simulink model "uas_sim"  (R2020b)
settings: Solver=VariableStepAuto  StartTime=0.0  StopTime=10.0  RelTol=1e-3  SampleTimeConstraint=STIndependent
undefined symbols (not defined in the file): Aircraft, datetime, datevec, Earth, Env, InitCond, WGS84
libraries: aerolibconvert2 x8, simulink x8, aerolibadyn x3, aerolibasang x3, aerolibtransform2 x2, aerolibatmos2 x1, sharedutil x1, aerolibbdyn x1, shared6dof x1, aerolibgravity2 x1
(part 2 of 2)

== system uas_sim/Flight Management Unit/Sensor Models/IMU/Accelerometer ==
  Body Accel [m/s/s] : Inport  PortDimensions=3
  Gravitational Accel in Body Frame [m/s/s] : Inport  Port=2  PortDimensions=3
  Add : Sum  Inputs=+++
  Band-Limited White Noise : simulink/Sources/Band-Limited White Noise  Cov=Aircraft.Sensors.Imu.Accel.noise_mps2  Ts=0.1  seed=[23341]
  Constant : Constant  Value=Aircraft.Sensors.Imu.Accel.bias_mps2  VectorParams1D=off
  Constant1 : Constant  Value=Aircraft.Sensors.Imu.Accel.scale_factor
  Product : Product  Multiplication=Matrix(*)
  Reshape : Reshape  OutputDimensionality=Column vector (2-D)
  Reshape1 : Reshape  OutputDimensionality=Column vector (2-D)
  Reshape2 : Reshape
  Saturation : Saturate  UpperLimit=Aircraft.Sensors.Imu.Accel.upper_limit_mps2  LowerLimit=Aircraft.Sensors.Imu.Accel.lower_limit_mps2
  Subtract : Sum  Inputs=+-
  Accelerometer [m/s/s] : Outport  PortDimensions=3
  wires:
  Add/1 -> Saturation/1
  Band-Limited White Noise/1 -> Add/1
  Product/1 -> Add/3
  Constant/1 -> Add/2
  Constant1/1 -> Product/1
  Subtract/1 -> Product/2
  Reshape/1 -> Subtract/2
  Gravitational Accel in Body Frame [m/s/s]/1 -> Reshape/1
  Reshape1/1 -> Subtract/1
  Body Accel [m/s/s]/1 -> Reshape1/1
  Saturation/1 -> Reshape2/1
  Reshape2/1 -> Accelerometer [m/s/s]/1

== system uas_sim/Flight Management Unit/Sensor Models/IMU/Gyro ==
  Body Rotational Rate [rad/s] : Inport  PortDimensions=3
  Body Accel [m/s/s] : Inport  Port=2  PortDimensions=3
  Add1 : Sum  Inputs=++++
  Band-Limited White Noise : simulink/Sources/Band-Limited White Noise  Cov=Aircraft.Sensors.Imu.Gyro.noise_radps  Ts=0.1  seed=[23341]  VectorParams1D=off
  Constant1 : Constant  Value=Aircraft.Sensors.Imu.Gyro.bias_radps  VectorParams1D=off
  Constant2 : Constant  Value=Aircraft.Sensors.Imu.Gyro.accel_sens_radps
  Constant3 : Constant  Value=Aircraft.Sensors.Imu.Gyro.scale_factor  VectorParams1D=off
  Product : Product
  Product1 : Product  Multiplication=Matrix(*)
  Reshape : Reshape  OutputDimensionality=Column vector (2-D)
  Reshape1 : Reshape  OutputDimensionality=Column vector (2-D)
  Reshape2 : Reshape
  Saturation : Saturate  UpperLimit=Aircraft.Sensors.Imu.Gyro.upper_limit_radps  LowerLimit=Aircraft.Sensors.Imu.Gyro.lower_limit_radps
  Gyro [rad/s] : Outport  PortDimensions=3
  wires:
  Constant3/1 -> Product1/1
  Constant2/1 -> Product/1
  Add1/1 -> Saturation/1
  Constant1/1 -> Add1/3
  Product1/1 -> Add1/4
  Band-Limited White Noise/1 -> Add1/2
  Body Rotational Rate [rad/s]/1 -> Reshape/1
  Reshape/1 -> Product1/2
  Body Accel [m/s/s]/1 -> Product/2
  Product/1 -> Reshape1/1
  Reshape1/1 -> Add1/1
  Reshape2/1 -> Gyro [rad/s]/1
  Saturation/1 -> Reshape2/1

== system uas_sim/Flight Management Unit/Sensor Models/IMU/Magnetometer ==
  Body Magnetic Field [uT] : Inport  PortDimensions=3
  Add2 : Sum  Inputs=+++
  Band-Limited White Noise : simulink/Sources/Band-Limited White Noise  Cov=Aircraft.Sensors.Imu.Mag.noise_ut  Ts=0.1  seed=[23341]
  Constant1 : Constant  Value=Aircraft.Sensors.Imu.Mag.scale_factor  VectorParams1D=off
  Constant2 : Constant  Value=Aircraft.Sensors.Imu.Mag.bias_ut
  Product : Product  Multiplication=Matrix(*)
  Reshape : Reshape  OutputDimensionality=Column vector (2-D)
  Reshape1 : Reshape
  Saturation : Saturate  UpperLimit=Aircraft.Sensors.Imu.Mag.upper_limit_ut  LowerLimit=Aircraft.Sensors.Imu.Mag.lower_limit_ut
  Magnetometer [uT] : Outport  PortDimensions=3
  wires:
  Body Magnetic Field [uT]/1 -> Reshape/1
  Band-Limited White Noise/1 -> Add2/1
  Add2/1 -> Saturation/1
  Constant2/1 -> Add2/2
  Constant1/1 -> Product/1
  Reshape/1 -> Product/2
  Saturation/1 -> Reshape1/1
  Reshape1/1 -> Magnetometer [uT]/1
  Product/1 -> Add2/3

== system uas_sim/Flight Management Unit/Vehicle Management System/Sensor Data Mapping/Air Data Mapping ==
  Virtual : Inport
  Bus Creator : BusCreator  Inputs=2  OutDataTypeStr=Bus: AirData
      settings: InheritFromInputs=off
  Bus Selector : BusSelector  OutputSignals=Static Pressure [Pa],Differential Pressure [Pa]
  Data Type Conversion1 : DataTypeConversion  OutDataTypeStr=single
  Data Type Conversion6 : DataTypeConversion  OutDataTypeStr=single
  Non-virtual : Outport  OutDataTypeStr=Bus: AirData
  wires:
  Virtual/1 -> Bus Selector/1
  Bus Creator/1 -> Non-virtual/1
  Bus Selector/2 -> Data Type Conversion1/1  "<Differential Pressure [Pa]>"
  Bus Selector/1 -> Data Type Conversion6/1  "<Static Pressure [Pa]>"
  Data Type Conversion6/1 -> Bus Creator/1  "static_pres_pa"
  Data Type Conversion1/1 -> Bus Creator/2  "diff_pres_pa"

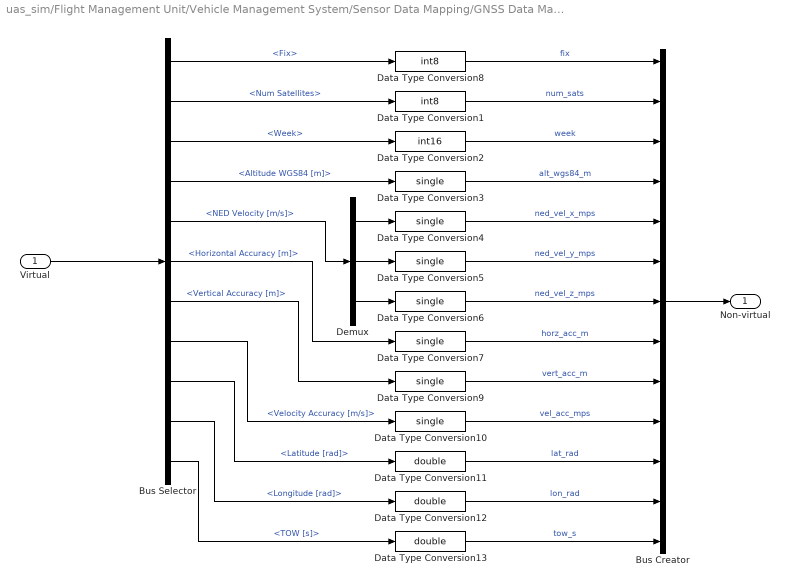
== system uas_sim/Flight Management Unit/Vehicle Management System/Sensor Data Mapping/GNSS Data Mapping ==
  Virtual : Inport
  Bus Creator : BusCreator  Inputs=13  OutDataTypeStr=Bus: GnssData
      settings: InheritFromInputs=off
  Bus Selector : BusSelector  OutputSignals=Fix,Num Satellites,Week,Altitude WGS84 [m],NED Velocity [m/s],Horizontal Accuracy [m],Vertical Accuracy [m],Velocity Accuracy [m/s],Latitude [rad],Longitude [rad],TOW [s]
  Data Type Conversion1 : DataTypeConversion  OutDataTypeStr=int8
  Data Type Conversion{3..7,9..10} (7 alike) : DataTypeConversion  OutDataTypeStr=single
  Data Type Conversion11 : DataTypeConversion  OutDataTypeStr=double
  Data Type Conversion12 : DataTypeConversion  OutDataTypeStr=double
  Data Type Conversion13 : DataTypeConversion  OutDataTypeStr=double
  Data Type Conversion2 : DataTypeConversion  OutDataTypeStr=int16
  Data Type Conversion8 : DataTypeConversion  OutDataTypeStr=int8
  Demux : Demux  Outputs=3
  Non-virtual : Outport  OutDataTypeStr=Bus: GnssData
  wires:
  Bus Creator/1 -> Non-virtual/1
  Virtual/1 -> Bus Selector/1
  Bus Selector/1 -> Data Type Conversion8/1  "<Fix>"
  Data Type Conversion8/1 -> Bus Creator/1  "fix"
  Bus Selector/2 -> Data Type Conversion1/1  "<Num Satellites>"
  Data Type Conversion1/1 -> Bus Creator/2  "num_sats"
  Data Type Conversion2/1 -> Bus Creator/3  "week"
  Bus Selector/3 -> Data Type Conversion2/1  "<Week>"
  Bus Selector/4 -> Data Type Conversion3/1  "<Altitude WGS84 [m]>"
  Data Type Conversion3/1 -> Bus Creator/4  "alt_wgs84_m"
  Demux/2 -> Data Type Conversion5/1
  Demux/1 -> Data Type Conversion4/1
  Demux/3 -> Data Type Conversion6/1
  Bus Selector/5 -> Demux/1  "<NED Velocity [m/s]>"
  Data Type Conversion4/1 -> Bus Creator/5  "ned_vel_x_mps"
  Data Type Conversion5/1 -> Bus Creator/6  "ned_vel_y_mps"
  Data Type Conversion6/1 -> Bus Creator/7  "ned_vel_z_mps"
  Data Type Conversion7/1 -> Bus Creator/8  "horz_acc_m"
  Bus Selector/6 -> Data Type Conversion7/1  "<Horizontal Accuracy [m]>"
  Data Type Conversion9/1 -> Bus Creator/9  "vert_acc_m"
  Data Type Conversion10/1 -> Bus Creator/10  "vel_acc_mps"
  Data Type Conversion11/1 -> Bus Creator/11  "lat_rad"
  Data Type Conversion12/1 -> Bus Creator/12  "lon_rad"
  Data Type Conversion13/1 -> Bus Creator/13  "tow_s"
  Bus Selector/11 -> Data Type Conversion13/1  "<TOW [s]>"
  Bus Selector/10 -> Data Type Conversion12/1  "<Longitude [rad]>"
  Bus Selector/9 -> Data Type Conversion11/1  "<Latitude [rad]>"
  Bus Selector/8 -> Data Type Conversion10/1  "<Velocity Accuracy [m/s]>"
  Bus Selector/7 -> Data Type Conversion9/1  "<Vertical Accuracy [m]>"

== system uas_sim/Flight Management Unit/Vehicle Management System/Sensor Data Mapping/IMU Data Mapping ==
  Virtual : Inport
  Bus Creator : BusCreator  Inputs=9  OutDataTypeStr=Bus: ImuData
      settings: InheritFromInputs=off
  Bus Selector : BusSelector  OutputSignals=Accelerometer [m/s/s],Gyro [rad/s],Magnetometer [uT]
  Data Type Conversion{1..9} (9 alike) : DataTypeConversion  OutDataTypeStr=single
  Demux : Demux  Outputs=3
  Demux1 : Demux  Outputs=3
  Demux2 : Demux  Outputs=3
  Non-virtual : Outport  OutDataTypeStr=Bus: ImuData
  wires:
  Virtual/1 -> Bus Selector/1
  Bus Creator/1 -> Non-virtual/1
  Demux/1 -> Data Type Conversion8/1
  Data Type Conversion8/1 -> Bus Creator/1  "accel_x_mps2"
  Demux/2 -> Data Type Conversion1/1
  Data Type Conversion1/1 -> Bus Creator/2  "accel_y_mps2"
  Demux/3 -> Data Type Conversion2/1
  Data Type Conversion2/1 -> Bus Creator/3  "accel_z_mps2"
  Data Type Conversion4/1 -> Bus Creator/6  "gyro_z_radps"
  Demux1/3 -> Data Type Conversion4/1
  Data Type Conversion3/1 -> Bus Creator/5  "gyro_y_radps"
  Demux1/2 -> Data Type Conversion3/1
  Data Type Conversion5/1 -> Bus Creator/4  "gyro_x_radps"
  Demux1/1 -> Data Type Conversion5/1
  Demux2/1 -> Data Type Conversion9/1
  Data Type Conversion9/1 -> Bus Creator/7  "mag_x_ut"
  Demux2/2 -> Data Type Conversion6/1
  Data Type Conversion6/1 -> Bus Creator/8  "mag_y_ut"
  Demux2/3 -> Data Type Conversion7/1
  Data Type Conversion7/1 -> Bus Creator/9  "mag_z-ut"
  Bus Selector/1 -> Demux/1  "<Accelerometer [m/s/s]>"
  Bus Selector/2 -> Demux1/1  "<Gyro [rad/s]>"
  Bus Selector/3 -> Demux2/1  "<Magnetometer [uT]>"

== system uas_sim/Vehicle/Forces and Moments/Aerodynamic/Aerodynamic Forces and Moments Coef Axis Variant ==
  Coef : Inport
  Dynamic Pressure [Pa] : Inport  Port=2
  Body Velocity [m/s] : Inport  Port=3
  Body Axis Coef : Subsystem  VariantControl=Aircraft.Aero.axis == 3
  Stability Axis Coef : Subsystem  VariantControl=Aircraft.Aero.axis == 2
  Wind Axis Coef : Subsystem  VariantControl=Aircraft.Aero.axis == 1
  Fxyz Mxyz : Outport

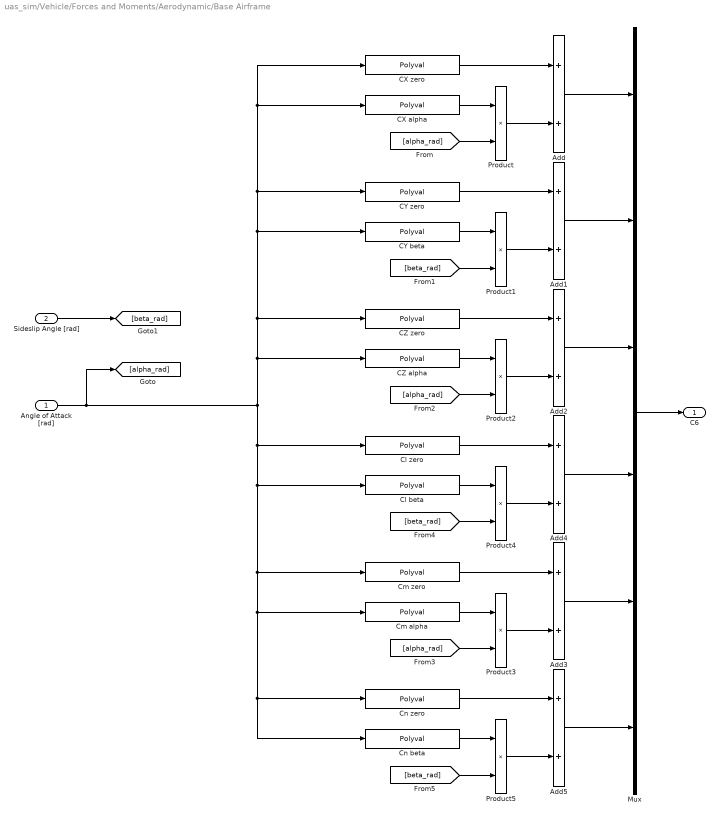
== system uas_sim/Vehicle/Forces and Moments/Aerodynamic/Base Airframe ==
  Angle of Attack [rad] : Inport
  Sideslip Angle [rad] : Inport  Port=2
  Add{,1..5} (6 alike) : Sum
  CX alpha : Polyval  Coefs=Aircraft.Aero.CX.alpha
  CX zero : Polyval  Coefs=Aircraft.Aero.CX.zero
  CY beta : Polyval  Coefs=Aircraft.Aero.CY.beta
  CY zero : Polyval  Coefs=Aircraft.Aero.CY.zero
  CZ alpha : Polyval  Coefs=Aircraft.Aero.CZ.alpha
  CZ zero : Polyval  Coefs=Aircraft.Aero.CZ.zero
  Cl beta : Polyval  Coefs=Aircraft.Aero.Cl.beta
  Cl zero : Polyval  Coefs=Aircraft.Aero.Cl.zero
  Cm alpha : Polyval  Coefs=Aircraft.Aero.Cm.alpha
  Cm zero : Polyval  Coefs=Aircraft.Aero.Cm.zero
  Cn beta : Polyval  Coefs=Aircraft.Aero.Cn.beta
  Cn zero : Polyval  Coefs=Aircraft.Aero.Cn.zero
  Mux : Mux  Inputs=6
  Product{,1..5} (6 alike) : Product
  C6 : Outport
  wires:
  Product/1 -> Add/2
  Add/1 -> Mux/1
  CX alpha/1 -> Product/1
  CX zero/1 -> Add/1
  Sideslip Angle [rad]/1 -> [beta_rad]
  [alpha_rad] -> Product/2
  Mux/1 -> C6/1
  [beta_rad] -> Product1/2
  CY zero/1 -> Add1/1
  CY beta/1 -> Product1/1
  Product1/1 -> Add1/2
  Add1/1 -> Mux/2
  CZ zero/1 -> Add2/1
  CZ alpha/1 -> Product2/1
  Add2/1 -> Mux/3
  Product2/1 -> Add2/2
  Product3/1 -> Add3/2
  Add3/1 -> Mux/5
  Cm alpha/1 -> Product3/1
  Cm zero/1 -> Add3/1
  [alpha_rad] -> Product2/2
  [alpha_rad] -> Product3/2
  Add4/1 -> Mux/4
  Product4/1 -> Add4/2
  Cl beta/1 -> Product4/1
  Cl zero/1 -> Add4/1
  [beta_rad] -> Product4/2
  [beta_rad] -> Product5/2
  Cn zero/1 -> Add5/1
  Cn beta/1 -> Product5/1
  Product5/1 -> Add5/2
  Add5/1 -> Mux/6
  Angle of Attack [rad]/1 -> [alpha_rad], Cl zero/1, Cl beta/1, Cm zero/1, Cm alpha/1, Cn zero/1, Cn beta/1, CZ alpha/1, CZ zero/1, CY beta/1, CY zero/1, CX alpha/1, CX zero/1

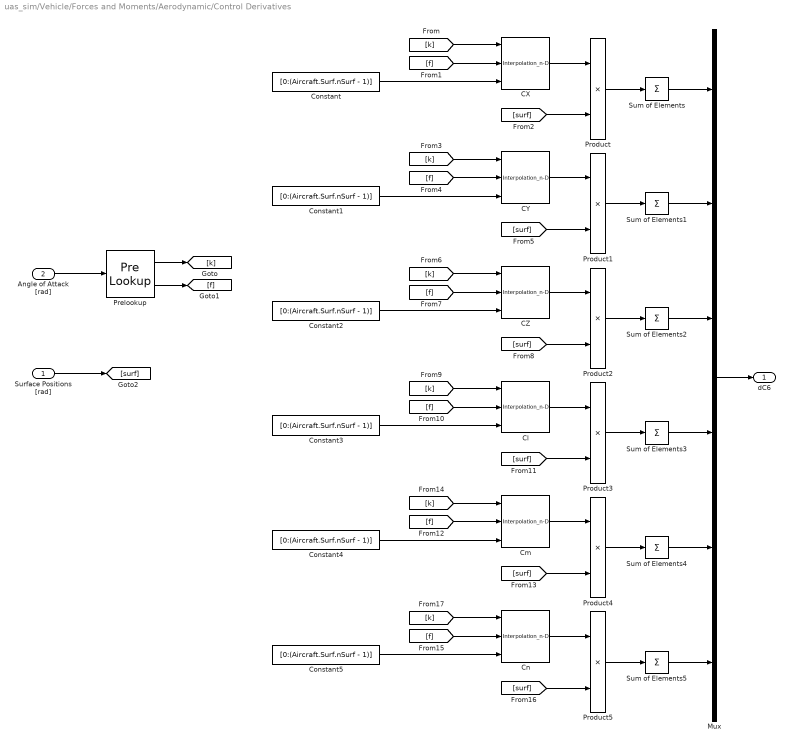
== system uas_sim/Vehicle/Forces and Moments/Aerodynamic/Control Derivatives ==
  Surface Positions [rad] : Inport
  Angle of Attack [rad] : Inport  Port=2
  CX : Interpolation_n-D  Table=Aircraft.Aero.CX.surf  DiagnosticForOutOfRangeInput=Warning  NumSelectionDims=1  InternalRulePriority=Speed
      settings: InputPortMap=u0,u1,u2
  CY : Interpolation_n-D  Table=Aircraft.Aero.CY.surf  DiagnosticForOutOfRangeInput=Warning  NumSelectionDims=1  InternalRulePriority=Speed
      settings: InputPortMap=u0,u1,u2
  CZ : Interpolation_n-D  Table=Aircraft.Aero.CZ.surf  DiagnosticForOutOfRangeInput=Warning  NumSelectionDims=1  InternalRulePriority=Speed
      settings: InputPortMap=u0,u1,u2
  Cl : Interpolation_n-D  Table=Aircraft.Aero.Cl.surf  DiagnosticForOutOfRangeInput=Warning  NumSelectionDims=1  InternalRulePriority=Speed
      settings: InputPortMap=u0,u1,u2
  Cm : Interpolation_n-D  Table=Aircraft.Aero.Cm.surf  DiagnosticForOutOfRangeInput=Warning  NumSelectionDims=1  InternalRulePriority=Speed
      settings: InputPortMap=u0,u1,u2
  Cn : Interpolation_n-D  Table=Aircraft.Aero.Cn.surf  DiagnosticForOutOfRangeInput=Warning  NumSelectionDims=1  InternalRulePriority=Speed
      settings: InputPortMap=u0,u1,u2
  Constant{,1..5} (6 alike) : Constant  Value=[0:(Aircraft.Surf.nSurf - 1)]
  Mux : Mux  Inputs=6
  Prelookup : PreLookup  BreakpointsData=Aircraft.Aero.CntrlEff.alpha  ExtrapMethod=Linear
  Product{,1..5} (6 alike) : Product
  Sum of Elements{,1..5} (6 alike) : Sum  Inputs=+
  dC6 : Outport
  wires:
  [k] -> Cm/1
  CY/1 -> Product1/1
  [f] -> Cn/2
  Product5/1 -> Sum of Elements5/1
  [surf] -> Product5/2
  Constant4/1 -> Cm/3
  Sum of Elements1/1 -> Mux/2
  [k] -> Cn/1
  Sum of Elements5/1 -> Mux/6
  Constant3/1 -> Cl/3
  [surf] -> Product3/2
  [k] -> Cl/1
  [f] -> Cl/2
  Constant2/1 -> CZ/3
  [k] -> CZ/1
  [surf] -> Product2/2
  Cl/1 -> Product3/1
  CZ/1 -> Product2/1
  Product2/1 -> Sum of Elements2/1
  Product3/1 -> Sum of Elements3/1
  Product1/1 -> Sum of Elements1/1
  Product/1 -> Sum of Elements/1
  [k] -> CY/1
  [f] -> CY/2
  Constant1/1 -> CY/3
  Constant/1 -> CX/3
  Cm/1 -> Product4/1
  [k] -> CX/1
  [surf] -> Product/2
  Prelookup/2 -> [f]
  Mux/1 -> dC6/1
  Prelookup/1 -> [k]
  Product4/1 -> Sum of Elements4/1
  Cn/1 -> Product5/1
  Angle of Attack [rad]/1 -> Prelookup/1
  Surface Positions [rad]/1 -> [surf]
  [f] -> CZ/2
  [f] -> Cm/2
  Sum of Elements2/1 -> Mux/3
  CX/1 -> Product/1
  [f] -> CX/2
  Constant5/1 -> Cn/3
  [surf] -> Product4/2
  Sum of Elements/1 -> Mux/1
  Sum of Elements4/1 -> Mux/5
  [surf] -> Product1/2
  Sum of Elements3/1 -> Mux/4

== system uas_sim/Vehicle/Forces and Moments/Aerodynamic/Dynamic Derivatives ==
  note: Divide by zero protection
  Airspeed [m/s] : Inport
  Body Rotational Rate [rad/s] : Inport  Port=2
  Angle of Attack [rad] : Inport  Port=3
  Add : Sum  Inputs=+++
  Constant : Constant  Value=Aircraft.Geom.b_m
  Constant1 : Constant  Value=Aircraft.Geom.c_m
  Constant2 : Constant  Value=Aircraft.Geom.b_m
  Demux : Demux  Outputs=3
  Divide : Product  Inputs=*/
  Gain : Gain  Gain=2
  Mux : Mux  Inputs=3
  Pitch Rate : Subsystem
  Product : Product
  Roll Rate : Subsystem
  Saturation : Saturate  UpperLimit=inf  LowerLimit=1e-3
  Yaw Rate : Subsystem
  dC6 : Outport
  wires:
  Constant/1 -> Mux/1
  Body Rotational Rate [rad/s]/1 -> Product/1
  Mux/1 -> Product/2
  Airspeed [m/s]/1 -> Gain/1
  Gain/1 -> Saturation/1
  Product/1 -> Divide/1
  Saturation/1 -> Divide/2
  Divide/1 -> Demux/1
  Demux/1 -> Roll Rate/2(p_hat)
  Demux/2 -> Pitch Rate/2(q_hat)
  Demux/3 -> Yaw Rate/2(r_hat)
  Angle of Attack [rad]/1 -> Yaw Rate/1(Angle of Attack [rad]), Pitch Rate/1(Angle of Attack [rad]), Roll Rate/1(Angle of Attack [rad])
  Roll Rate/1(dC6) -> Add/1
  Pitch Rate/1(dC6) -> Add/2
  Yaw Rate/1(dC6) -> Add/3
  Constant2/1 -> Mux/3
  Constant1/1 -> Mux/2
  Add/1 -> dC6/1

== system uas_sim/Vehicle/Forces and Moments/Propulsive/Motor ==
  note: RPM to rad/s
  Voltage [V] : Inport
  Motor Rotation Rate [rad/s] : Inport  Port=2
  Constant : Constant  Value=Aircraft.Motor.kv
  Constant1 : Constant  Value=Aircraft.Motor.io
  Divide : Product  Inputs=*/
  Divide2 : Product  Inputs=*/
  Gain : Gain  Gain=1/Aircraft.Motor.r
  Gain2 : Gain  Gain=2 * pi / 60
  Subtract : Sum  Inputs=+-
  Subtract1 : Sum  Inputs=+-
  Torque [N-m] : Outport
  wires:
  Gain2/1 -> [KvSI], Divide/2
  [KvSI] -> Divide2/2
  Constant1/1 -> Subtract1/2
  Motor Rotation Rate [rad/s]/1 -> Divide/1
  Divide/1 -> Subtract/2
  Constant/1 -> Gain2/1
  Gain/1 -> Subtract1/1
  Subtract1/1 -> Divide2/1
  Voltage [V]/1 -> Subtract/1
  Divide2/1 -> Torque [N-m]/1
  Subtract/1 -> Gain/1

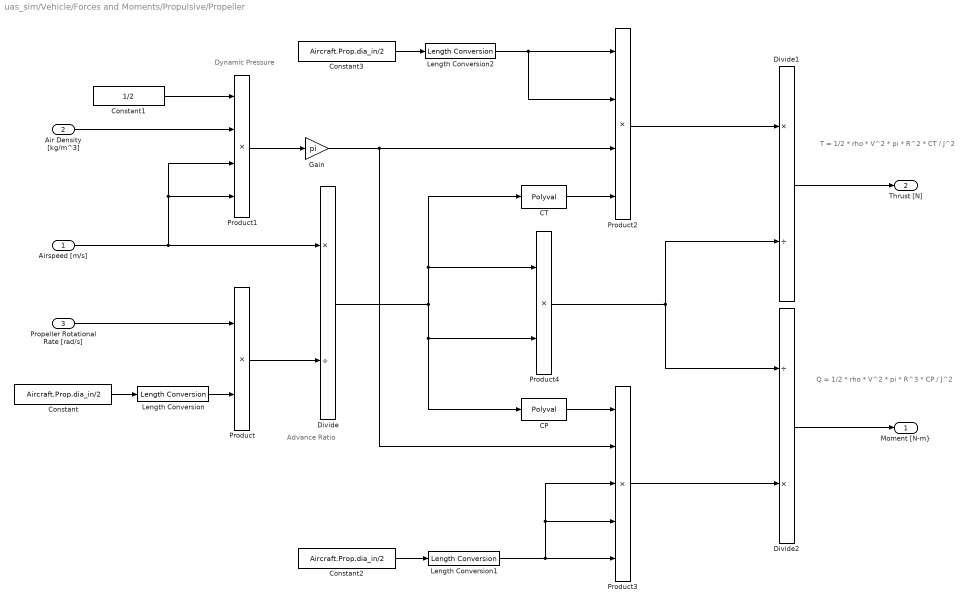
== system uas_sim/Vehicle/Forces and Moments/Propulsive/Propeller ==
  note: Dynamic Pressure
  note: Q = 1/2 * rho * V^2 * pi * R^3 * CP / J^2
  note: T = 1/2 * rho * V^2 * pi * R^2 * CT / J^2
  note: Advance Ratio
  Airspeed [m/s] : Inport
  Air Density [kg/m^3] : Inport  Port=2
  Propeller Rotational Rate [rad/s] : Inport  Port=3
  CP : Polyval  Coefs=Aircraft.prop.cp
  CT : Polyval  Coefs=Aircraft.prop.ct
  Constant : Constant  Value=Aircraft.Prop.dia_in/2
  Constant1 : Constant  Value=1/2
  Constant2 : Constant  Value=Aircraft.Prop.dia_in/2
  Constant3 : Constant  Value=Aircraft.Prop.dia_in/2
  Divide : Product  Inputs=*/
  Divide1 : Product  Inputs=*/
  Divide2 : Product  Inputs=/*
  Gain : Gain  Gain=pi
  Length Conversion : aerolibconvert2/Length Conversion  IU=in  OU=m
  Length Conversion1 : aerolibconvert2/Length Conversion  IU=in  OU=m
  Length Conversion2 : aerolibconvert2/Length Conversion  IU=in  OU=m
  Product : Product
  Product1 : Product  Inputs=4
  Product2 : Product  Inputs=4
  Product3 : Product  Inputs=5
  Product4 : Product
  "Moment [N-m}" : Outport
  Thrust [N] : Outport  Port=2
  wires:
  Divide2/1 -> "Moment [N-m}"/1
  Length Conversion/1 -> Product/2
  Product4/1 -> Divide2/1, Divide1/2
  Constant2/1 -> Length Conversion1/1
  Airspeed [m/s]/1 -> Divide/1, Product1/4, Product1/3
  Propeller Rotational Rate [rad/s]/1 -> Product/1
  Length Conversion1/1 -> Product3/4, Product3/3, Product3/5
  Product1/1 -> Gain/1
  Gain/1 -> Product3/2, Product2/3
  Air Density [kg/m^3]/1 -> Product1/2
  Divide1/1 -> Thrust [N]/1
  Product3/1 -> Divide2/2
  Constant1/1 -> Product1/1
  CP/1 -> Product3/1
  CT/1 -> Product2/4
  Product2/1 -> Divide1/1
  Length Conversion2/1 -> Product2/2, Product2/1
  Constant/1 -> Length Conversion/1
  Constant3/1 -> Length Conversion2/1
  Divide/1 -> Product4/2, CP/1, Product4/1, CT/1
  Product/1 -> Divide/2

== system uas_sim/Vehicle/Forces and Moments/Aerodynamic/Aerodynamic Forces and Moments Coef Axis Variant/Body Axis Coef ==
  Coef : Inport
  Dynamic Pressure [Pa] : Inport  Port=2
  Body Velocity [m/s] : Inport  Port=3
  "Aerodynamic Forces and Moments " : aerolibadyn/Aerodynamic Forces and Moments   inputAxes=Body  outputForceAxes=Body  outputMomentAxes=Body  S=Aircraft.Geom.s_m2  b=Aircraft.Geom.b_m  cbar=Aircraft.Geom.c_m
  Constant : Constant  Value=Aircraft.Mass.cg_m
  Constant1 : Constant  Value=Aircraft.Geom.cp_m
  Mux : Mux  Inputs=2
  Terminator : Terminator
  Fxyz Mxyz : Outport
  wires:
  Mux/1 -> Fxyz Mxyz/1
  Constant1/1 -> "Aerodynamic Forces and Moments "/4
  Coef/1 -> "Aerodynamic Forces and Moments "/1
  Constant/1 -> "Aerodynamic Forces and Moments "/3
  "Aerodynamic Forces and Moments "/1 -> Mux/1
  "Aerodynamic Forces and Moments "/2 -> Mux/2
  Dynamic Pressure [Pa]/1 -> "Aerodynamic Forces and Moments "/2
  Body Velocity [m/s]/1 -> Terminator/1

== system uas_sim/Vehicle/Forces and Moments/Aerodynamic/Aerodynamic Forces and Moments Coef Axis Variant/Stability Axis Coef ==
  Coef : Inport
  Dynamic Pressure [Pa] : Inport  Port=2
  Body Velocity [m/s] : Inport  Port=3
  "Aerodynamic Forces and Moments " : aerolibadyn/Aerodynamic Forces and Moments   inputAxes=Stability  outputForceAxes=Body  outputMomentAxes=Body  S=Aircraft.Geom.s_m2  b=Aircraft.Geom.b_m  cbar=Aircraft.Geom.c_m
  Constant : Constant  Value=Aircraft.Mass.cg_m
  Constant1 : Constant  Value=Aircraft.Geom.cp_m
  Mux : Mux  Inputs=2
  Fxyz Mxyz : Outport
  wires:
  Dynamic Pressure [Pa]/1 -> "Aerodynamic Forces and Moments "/2
  "Aerodynamic Forces and Moments "/2 -> Mux/2
  "Aerodynamic Forces and Moments "/1 -> Mux/1
  Constant/1 -> "Aerodynamic Forces and Moments "/3
  Coef/1 -> "Aerodynamic Forces and Moments "/1
  Constant1/1 -> "Aerodynamic Forces and Moments "/4
  Mux/1 -> Fxyz Mxyz/1
  Body Velocity [m/s]/1 -> "Aerodynamic Forces and Moments "/5

== system uas_sim/Vehicle/Forces and Moments/Aerodynamic/Aerodynamic Forces and Moments Coef Axis Variant/Wind Axis Coef ==
  Coef : Inport
  Dynamic Pressure [Pa] : Inport  Port=2
  Body Velocity [m/s] : Inport  Port=3
  "Aerodynamic Forces and Moments " : aerolibadyn/Aerodynamic Forces and Moments   inputAxes=Wind  outputForceAxes=Body  outputMomentAxes=Body  S=Aircraft.Geom.s_m2  b=Aircraft.Geom.b_m  cbar=Aircraft.Geom.c_m
  Constant : Constant  Value=Aircraft.Mass.cg_m
  Constant1 : Constant  Value=Aircraft.Geom.cp_m
  Mux : Mux  Inputs=2
  Fxyz Mxyz : Outport
  wires:
  Dynamic Pressure [Pa]/1 -> "Aerodynamic Forces and Moments "/2
  Body Velocity [m/s]/1 -> "Aerodynamic Forces and Moments "/5
  "Aerodynamic Forces and Moments "/2 -> Mux/2
  "Aerodynamic Forces and Moments "/1 -> Mux/1
  Constant/1 -> "Aerodynamic Forces and Moments "/3
  Coef/1 -> "Aerodynamic Forces and Moments "/1
  Constant1/1 -> "Aerodynamic Forces and Moments "/4
  Mux/1 -> Fxyz Mxyz/1

== system uas_sim/Vehicle/Forces and Moments/Aerodynamic/Dynamic Derivatives/Pitch Rate ==
  Angle of Attack [rad] : Inport
  q_hat : Inport  Port=2
  CX q : Polyval  Coefs=Aircraft.Aero.CX.q
  CZ q : Polyval  Coefs=Aircraft.Aero.CZ.q
  Cm q : Polyval  Coefs=Aircraft.Aero.Cm.q
  Constant1 : Constant  Value=0
  Constant2 : Constant  Value=0
  Constant4 : Constant  Value=0
  Mux : Mux  Inputs=6
  Product : Product
  Product1 : Product
  Product2 : Product
  dC6 : Outport
  wires:
  Mux/1 -> dC6/1
  Constant1/1 -> Mux/2
  Product2/1 -> Mux/1
  Constant4/1 -> Mux/6
  Constant2/1 -> Mux/4
  Product/1 -> Mux/3
  Product1/1 -> Mux/5
  q_hat/1 -> Product2/2, Product1/2, Product/2
  CZ q/1 -> Product/1
  CX q/1 -> Product2/1
  Cm q/1 -> Product1/1
  Angle of Attack [rad]/1 -> CX q/1, Cm q/1, CZ q/1

== system uas_sim/Vehicle/Forces and Moments/Aerodynamic/Dynamic Derivatives/Roll Rate ==
  Angle of Attack [rad] : Inport
  p_hat : Inport  Port=2
  CY p : Polyval  Coefs=Aircraft.Aero.CY.p
  Cl p : Polyval  Coefs=Aircraft.Aero.Cl.p
  Cn p : Polyval  Coefs=Aircraft.Aero.Cn.p
  Constant : Constant  Value=0
  Constant2 : Constant  Value=0
  Constant4 : Constant  Value=0
  Mux : Mux  Inputs=6
  Product : Product
  Product1 : Product
  Product2 : Product
  dC6 : Outport
  wires:
  Product1/1 -> Mux/4
  Product2/1 -> Mux/6
  Constant/1 -> Mux/1
  Mux/1 -> dC6/1
  Product/1 -> Mux/2
  CY p/1 -> Product/1
  Cl p/1 -> Product1/1
  Constant2/1 -> Mux/3
  Constant4/1 -> Mux/5
  p_hat/1 -> Product2/2, Product1/2, Product/2
  Cn p/1 -> Product2/1
  Angle of Attack [rad]/1 -> Cn p/1, CY p/1, Cl p/1

== system uas_sim/Vehicle/Forces and Moments/Aerodynamic/Dynamic Derivatives/Yaw Rate ==
  Angle of Attack [rad] : Inport
  r_hat : Inport  Port=2
  CY r : Polyval  Coefs=Aircraft.Aero.CY.r
  Cl r : Polyval  Coefs=Aircraft.Aero.Cl.r
  Cn r : Polyval  Coefs=Aircraft.Aero.Cn.r
  Constant : Constant  Value=0
  Constant2 : Constant  Value=0
  Constant4 : Constant  Value=0
  Mux : Mux  Inputs=6
  Product : Product
  Product1 : Product
  Product2 : Product
  dC6 : Outport
  wires:
  r_hat/1 -> Product2/2, Product1/2, Product/2
  Mux/1 -> dC6/1
  CY r/1 -> Product/1
  Constant/1 -> Mux/1
  Product2/1 -> Mux/6
  Product/1 -> Mux/2
  Cl r/1 -> Product1/1
  Constant2/1 -> Mux/3
  Product1/1 -> Mux/4
  Constant4/1 -> Mux/5
  Cn r/1 -> Product2/1
  Angle of Attack [rad]/1 -> Cn r/1, CY r/1, Cl r/1

== matlab function uas_sim/Vehicle/Vehicle Model/MATLAB Function ==
  data: ang input; ret output
function ret  = constrain360(ang)
%Constrain360 Converts a +/-180 value to a 0 - 360 value
ret = fmod(ang, 360);
if ret < 0
    ret = ret + 360;
end

end

== matlab function uas_sim/Flight Management Unit/Sensor Models/GNSS/Triggered Subsystem/MATLAB Function ==
  data: year input; month input; mday input; hour input; minute input; second input; gnss_week output; sim_clock input; gnss_tow output
function [gnss_week, gnss_tow] = GnssWeekAndTime(year, month, mday, hour, minute, second, sim_clock)

JAN61980 = 44244;
JAN11901 = 15385;
SEC_PER_DAY = 86400.0;

month_day = [
    0, 31, 59, 90, 120, 151, 181, 212, 243, 273, 304, 334;
    0, 31, 60, 91, 121, 152, 182, 213, 244, 274, 305, 335
];

second = second + sim_clock;
leap = (mod(year,4) == 0);
yday = month_day(leap + 1, month) + mday;
mjd = ((year - 1901) / 4) * 1461 + mod((year - 1901), 4) * 365 + yday - 1 + JAN11901;
fmjd = ((second / 60.0 + minute) / 60.0 + hour) / 24.0;
gnss_week = floor((mjd - JAN61980) / 7);
gnss_tow = ((mjd - JAN61980) - gnss_week * 7 + fmjd) * SEC_PER_DAY;
